simulink model "VC_TakeColorPicturesAndSave"  (R2016b)
settings: Solver=ode45  StartTime=0.0  StopTime=inf  RelTol=1e-3  EnableMultiTasking=on
undefined symbols (not defined in the file or in its folder): IsPositionTracked, IsSkeletonTracked, JointDepthIndices, JointImageIndices, JointTrackingState, JointWorldCoordinates, none, PositionDepthIndices, PositionImageIndices, PositionWorldCoordinates, SegmentationData, SkeletonTrackingID, videoinput
libraries: visionsinks x4, imaqlib x2, simulink x1
settings Model: Creator=jcpinto  LastModifiedBy=Alexandra
settings DataIOCC: LimitDataPoints=on  SaveFormat=Array  SignalLoggingSaveFormat=ModelDataLogs
settings OptimizationCC: ExpressionDepthLimit=2147483647  LifeSpan=inf
settings DebuggingCC: UnderspecifiedInitializationDetection=Classic  MergeDetectMultiDrivingBlocksExec=none  SolverPrmCheckMsg=warning  FcnCallInpInsideContextMsg=warning  AllowSymbolicDim=off  StateNameClashWarn=warning  SFUnexpectedBacktrackingDiag=warning  SFNoUnconditionalDefaultTransitionDiag=warning  SFExecutionAtInitializationDiag=none
settings HardwareCC: ProdBitPerPointer=32  ProdBitPerSizeT=32  ProdBitPerPtrDiffT=32  ProdLargestAtomicFloat=None  ProdIntDivRoundTo=Undefined  ProdEndianess=Unspecified  ProdWordSize=32  ProdHWDeviceType=32-bit Generic
settings ModelReferenceCC: PropagateSignalLabelsOutOfModel=off
settings GRTTargetCC: TargetLangStandard=C89/C90 (ANSI)  GeneratePreprocessorConditionals=Disable all  CombineOutputUpdateFcns=off  GRTInterface=on
settings ConfigComp: CovMetricSettings=dw  CovHtmlReporting=on  CovSaveCumulativeToWorkspaceVar=on  CovSaveSingleToWorkspaceVar=on  CovExternalEMLEnable=off  CovSFcnEnable=off

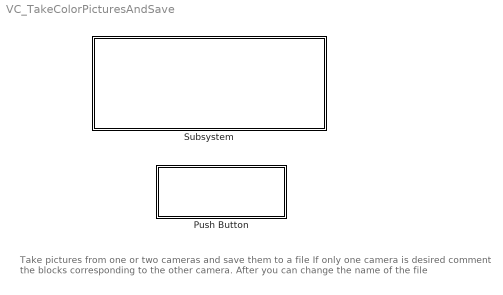
== system VC_TakeColorPicturesAndSave ==
  note: Take pictures from one or two cameras and save them to a file
      | If only one camera is desired comment the blocks corresponding to the other camera. After you can change the name of the file
  Push Button : Subsystem  DialogController=hmiCreateDDGDialog  IsWebBlock=on  mask(MWDashboardBlock){webBlockId=ec4db6c9-9411-4fe6-83e0-66052ec15a4a, webBlockType=pushbutton, ShowInLibBrwoser=on, ShowInitialText=on, HMISrcModelName=VC_TakeColorPicturesAndSave}
      mask prompts: webBlockId "WebBlock Id"; webBlockType "WebBlock Type"; HMISrcModelName "Source Model"
      mask Help: helpview([docroot '/mapfiles/simulink.map'], 'hmi_push_button')
      mask Display:
      | model = bdroot(gcb);
      | if strcmp(get_param(model,'BlockDiagramType'), 'library')
      |     image([(matlabroot) '/toolbox/simulink/hmi/icons/PushButton.png']);
      | end
  Subsystem : Subsystem
      mask Display:
      | disp('Take a pair of colour pictures and save\n\n\n\n')
      | disp('\n\n\n ')
      | disp('Computer Vision')
      | 
      | disp('\n\nACCAII/DEM/IST/UL')

== system VC_TakeColorPicturesAndSave/Push Button ==

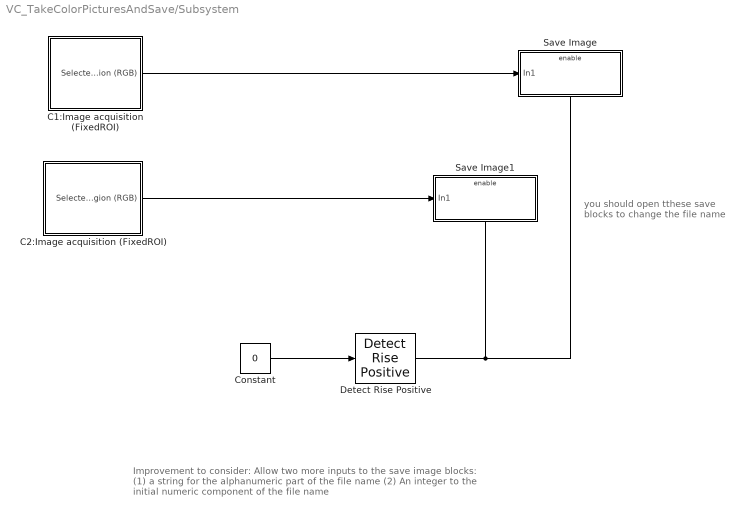
== system VC_TakeColorPicturesAndSave/Subsystem ==
  note: Improvement to consider:
      |
      | Allow two more inputs to the save image blocks:
      |      (1) a string for the alphanumeric part of the file name
      |      (2) An integer to the initial numeric component of the file name
  note: you should open tthese save blocks to change the file name
  C1:Image acquisition (FixedROI) : Subsystem
  C2:Image acquisition (FixedROI) : Subsystem
  Constant : Constant  Value=0  OutDataTypeStr=boolean
  Detect Rise Positive : simulink/Logic and Bit Operations/Detect Rise Positive  vinit=0  InputProcessing=Inherited  OutDataTypeStr=uint8
  Save Image : Subsystem  TreatAsAtomicUnit=on
  Save Image1 : Subsystem  TreatAsAtomicUnit=on
  wires:
  C1:Image acquisition (FixedROI)/1(Selected region (RGB)) -> Save Image/1(In1)
  Detect Rise Positive/1 -> Save Image1/Enable, Save Image/Enable
  C2:Image acquisition (FixedROI)/1(Selected region (RGB)) -> Save Image1/1(In1)
  Constant/1 -> Detect Rise Positive/1

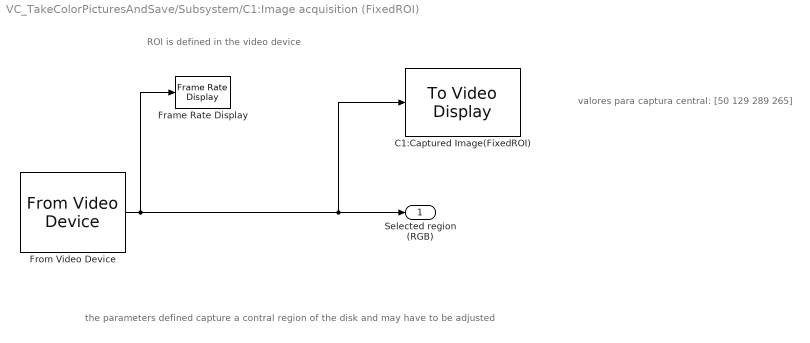
== system VC_TakeColorPicturesAndSave/Subsystem/C1:Image acquisition (FixedROI) ==
  note: valores para captura central: [50 129 289 265]
  note: the parameters defined capture a contral region of the disk and may have to be adjusted
  note: ROI is defined in the video device
  C1:Captured Image(FixedROI) : visionsinks/To Video Display  windowSizeMode=True size (1:1)  openAtMdlStart=on  fullScreen=off  videoWindowX=1122  videoWindowY=43  saveWindowSize=off  videoWindowWidth=320  videoWindowHeight=240  inputColorFormat=RGB  inputType=Obsolete  imagePorts=One multidimensional signal  OutputDevice=On-screen video monitor  dataOrg=Column-major  isWindowOpen=off
  Frame Rate Display : visionsinks/Frame Rate Display  UpdateRate=4
  From Video Device : imaqlib/From Video Device  DeviceMenu=winvideo 1 (USB2.0 PC CAMERA)  Device=winvideo 1 (USB2.0 PC CAMERA)  ObjConstructor=videoinput('winvideo', 1)  VideoFormatMenu=YUY2_320x240  VideoFormat=YUY2_320x240  VideoSource=input1  ROIPosition=[0 0 240 320]  EnableHWTrigger=off  TriggerConfiguration=none/none  SampleTime=1/30  OutputPortsMode=One multidimensional signal  DataType=single  CanDoHWTrigger=no  ReturnedColorSpace=YCbCr  BlockHandle=2078.0001  ROIWidth=320  ROIHeight=240  ROIColumn=0  ROIRow=0  EngXMLPath=C:\Program Files\MATLAB\R2016b\toolbox\imaq\imaq\private  DevXMLPath=C:\ProgramData\MATLAB\SupportPackages\R2016b\toolbox\imaq\supportpackages\genericvideo\adaptor\win64  EngLibPath=C:\Program Files\MATLAB\R2016b\toolbox\imaq\imaqblks\imaqmex\win64  ColorSpace=YCbCr  BayerSensorAlignment=grbg  AllMetadata=IsPositionTracked;IsSkeletonTracked;JointDepthIndices;JointImageIndices;JointTrackingState;JointWorldCoordinates;PositionDepthIndices;PositionImageIndices;PositionWorldCoordinates;SegmentationData;SkeletonTrackingID
  Selected region (RGB) : Outport
  wires:
  From Video Device/1 -> Frame Rate Display/1, C1:Captured Image(FixedROI)/1, Selected region (RGB)/1

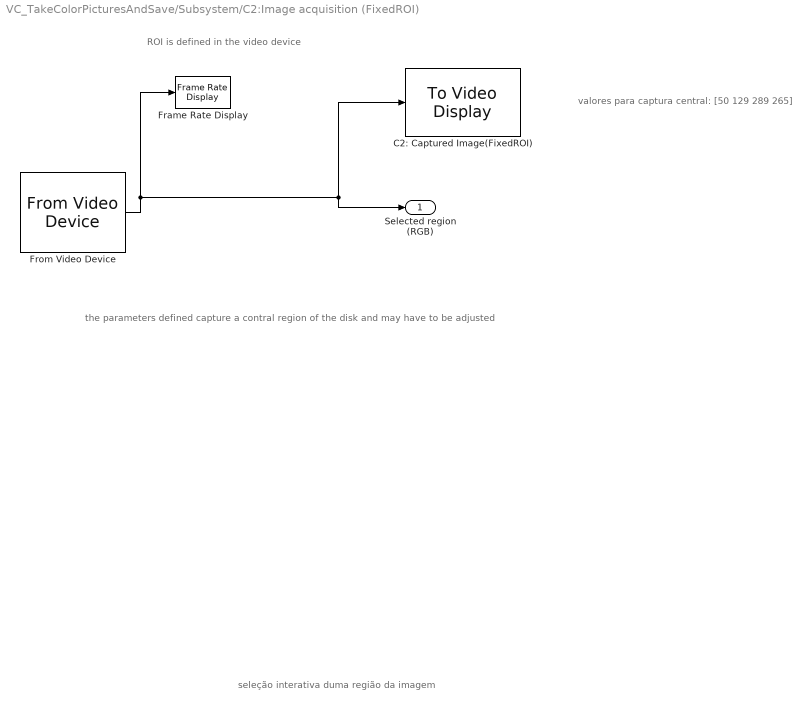
== system VC_TakeColorPicturesAndSave/Subsystem/C2:Image acquisition (FixedROI) ==
  note: valores para captura central: [50 129 289 265]
  note: the parameters defined capture a contral region of the disk and may have to be adjusted
  note: ROI is defined in the video device
  note: seleção interativa duma região da imagem
  C2: Captured Image(FixedROI) : visionsinks/To Video Display  windowSizeMode=True size (1:1)  openAtMdlStart=on  fullScreen=off  videoWindowX=1511  videoWindowY=34  saveWindowSize=off  videoWindowWidth=320  videoWindowHeight=240  inputColorFormat=RGB  inputType=Obsolete  imagePorts=One multidimensional signal  OutputDevice=On-screen video monitor  dataOrg=Column-major  isWindowOpen=off
  Frame Rate Display : visionsinks/Frame Rate Display  UpdateRate=4
  From Video Device : imaqlib/From Video Device  DeviceMenu=winvideo 1 (USB2.0 PC CAMERA)  Device=winvideo 2 (USB2.0 PC CAMERA)  ObjConstructor=videoinput('winvideo', 2)  VideoFormatMenu=YUY2_320x240  VideoFormat=YUY2_320x240  VideoSource=input1  ROIPosition=[0 0 240 320]  EnableHWTrigger=off  TriggerConfiguration=none/none  SampleTime=1/30  OutputPortsMode=One multidimensional signal  DataType=single  CanDoHWTrigger=no  ReturnedColorSpace=rgb  BlockHandle=2078.0001  ROIWidth=320  ROIHeight=240  ROIColumn=0  ROIRow=0  EngXMLPath=C:\Program Files\MATLAB\R2016b\toolbox\imaq\imaq\private  DevXMLPath=C:\ProgramData\MATLAB\SupportPackages\R2016b\toolbox\imaq\supportpackages\genericvideo\adaptor\win64  EngLibPath=C:\Program Files\MATLAB\R2016b\toolbox\imaq\imaqblks\imaqmex\win64  ColorSpace=rgb  BayerSensorAlignment=grbg  AllMetadata=IsPositionTracked;IsSkeletonTracked;JointDepthIndices;JointImageIndices;JointTrackingState;JointWorldCoordinates;PositionDepthIndices;PositionImageIndices;PositionWorldCoordinates;SegmentationData;SkeletonTrackingID
  Selected region (RGB) : Outport
  wires:
  From Video Device/1 -> Selected region (RGB)/1, C2: Captured Image(FixedROI)/1, Frame Rate Display/1

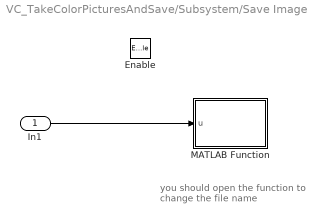
== system VC_TakeColorPicturesAndSave/Subsystem/Save Image ==
  note: you should open the function to change the file name
  In1 : Inport
  Enable : EnablePort
  MATLAB Function : MATLAB Function  TreatAsAtomicUnit=on
  wires:
  In1/1 -> MATLAB Function/1(u)

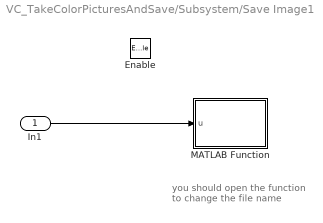
== system VC_TakeColorPicturesAndSave/Subsystem/Save Image1 ==
  note: you should open the function to change the file name
  In1 : Inport
  Enable : EnablePort
  MATLAB Function : MATLAB Function  TreatAsAtomicUnit=on
  wires:
  In1/1 -> MATLAB Function/1(u)

== matlab function VC_TakeColorPicturesAndSave/Subsystem/Save Image1/MATLAB Function ==
  data: u input
function fcn(u)
%#codegen

persistent n

if isempty(n)
   n = 0;
end
coder.extrinsic('imwrite');
coder.extrinsic('int2str');
%%%%%%%%%%%%%%%%%%%%%%%
n=n+1;
str = int2str(n);
 if n < 10
         imagename=['c2ima0' str '.jpg'];
       else
         imagename=['c2ima' str '.jpg'];
       end
imwrite(u,imagename,'jpg')

== matlab function VC_TakeColorPicturesAndSave/Subsystem/Save Image/MATLAB Function ==
  data: u input
function fcn(u)
%#codegen

persistent m

if isempty(m)
   m = 0;
end
coder.extrinsic('imwrite');
coder.extrinsic('int2str');
%%%%%%%%%%%%%%%%%%%%%%%
m=m+1;
str = int2str(m);
 if m < 10
         imagename=['c1ima0' str '.jpg'];
       else
         imagename=['c1ima' str '.jpg'];
       end
imwrite(u,imagename,'jpg')
